simulink model "pod_elevation_model"  (R2021b)
settings: Solver=ode45  StartTime=0.0  StopTime=20  RelTol=1e-3
values from neighbouring files (symbols this model uses):
  fric_gear_motor_pod_elevation = 0.23125*0.42    (= 0.097125)    [loading_project.m]
  ts3 = 10^-3    (= 0.001)    [loading_project.m]
libraries: simulink x3, dspsrcs4 x1
settings Model: Creator=noait  LastModifiedBy=noait

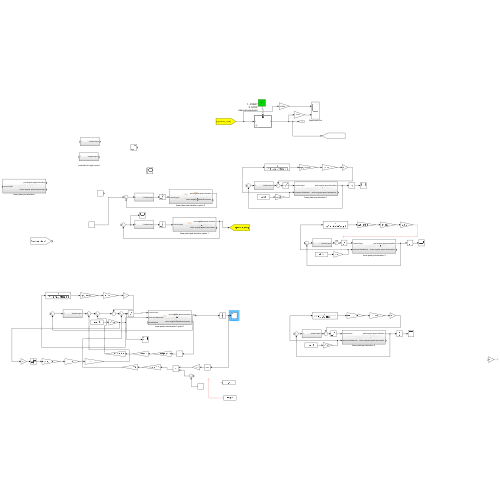
[thumbnail: Simulink's stored preview of the top-level diagram]
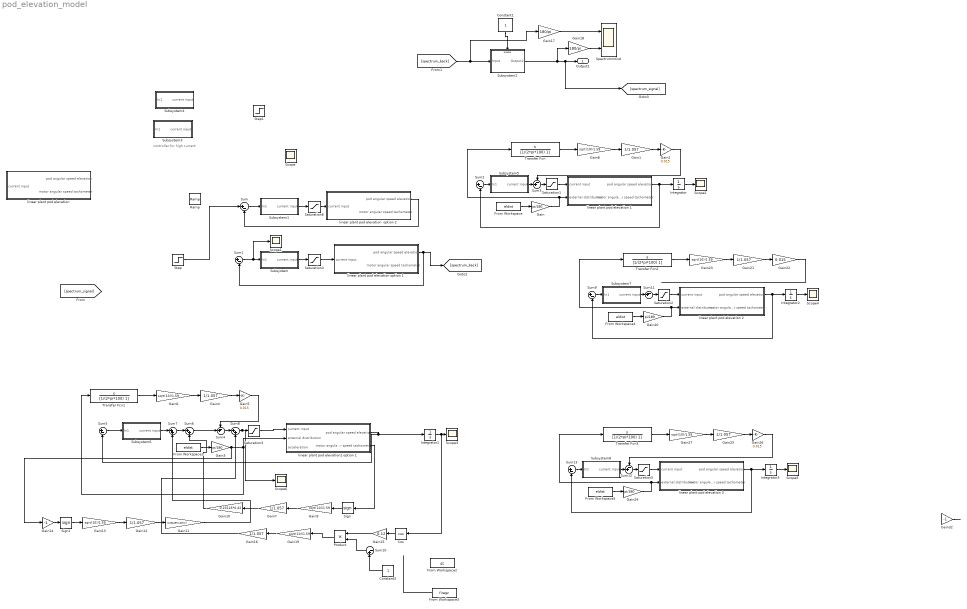
== system pod_elevation_model ==
  note: controller for high current
  Constant1 : Constant  OutDataTypeStr=boolean
      settings: AttributesFormatString=1 - START\n0 -STOP\ninternal spectrum
      settings: OpenFcn=|
      | if get_param(gcbh,'value')-48 set_param(gcbh,'value','0','backgroundcolor','red');
      | else set_param(gcbh,'value','1','backgroundcolor','green');
      | end
  Constant3 : Constant
  Cos : Trigonometry  Operator=cos
  From Workspace{,1,4..5} (4 alike) : FromWorkspace  VariableName=eldist  SampleTime=ts3/3  Interpolate=off  ZeroCross=off  OutputAfterFinalValue=Setting to zero
  From Workspace2 : FromWorkspace  VariableName=gz  SampleTime=ts3/3  Interpolate=off  ZeroCross=off  OutputAfterFinalValue=Setting to zero
  From Workspace3 : FromWorkspace  VariableName=firegz  SampleTime=ts3/9  Interpolate=off  ZeroCross=off  OutputAfterFinalValue=Setting to zero
  Gain{,3,20,24} (4 alike) : Gain  Gain=pi/180
  Gain{1,4,7,12,16,21,25} (7 alike) : Gain  Gain=1/1.057
  Gain10 : Gain  Gain=0.23125*0.42
  Gain11 : Gain  Gain=0.23125*0.42*0.7
  Gain{6,8..9,13,19,23,27} (7 alike) : Gain  Gain=sqrt(10)/1.59
  Gain14 : Gain  Gain=-1
  Gain15 : Gain  Gain=0.12
  Gain17 : Gain  Gain=180/pi
  Gain18 : Gain  Gain=180/pi
  Gain{2,5,22,26} (4 alike) : Gain  Gain=0.015
  Gain32 : Gain  Gain=-1
  Integrator{,1..3} (4 alike) : Integrator
  Product : Product
  Ramp : simulink/Sources/Ramp  slope=1  start=0  InitialOutput=0
  Saturation{1..2,4..5} (4 alike) : Saturate  UpperLimit=11.933*sqrt(10)/1.59  LowerLimit=-11.933*sqrt(10)/1.59  ZeroCross=off
  Saturation3 : Saturate  UpperLimit=11.933*sqrt(10)/1.59  LowerLimit=-11.933*sqrt(10)/1.59
  Saturation6 : Saturate  UpperLimit=11.933*sqrt(10)*0.5/(1.59*0.52)  LowerLimit=-11.933*sqrt(10)*0.5/(1.59*0.52)  ZeroCross=off
  Scope : Scope  NumInputPorts=2
  Scope{1..6} (6 alike) : Scope
  Sign : Signum
  Sign1 : Signum
  SpectrumInOut : Scope  NumInputPorts=2
  Step : Step  SampleTime=0  ZeroCross=off
  Step1 : Step  After=22  SampleTime=0
  Subsystem : Subsystem
  Subsystem1 : Subsystem
  Subsystem2 : Subsystem  mask{GAIN=0.1%2*pi/180%0.5*pi/180, InitFreq=1, TargetTime=500, FreqAtTime=500}
      mask prompts: InitFreq "INITIAL FREQUENCY"; TargetTime "Target Time"; FreqAtTime "Frequency at Time"
  Subsystem3 : Subsystem
  Subsystem4 : Subsystem
  Subsystem5 : Subsystem
  Subsystem6 : Subsystem
  Subsystem7 : Subsystem
  Subsystem8 : Subsystem
  Sum{,1..2,5,9,13} (6 alike) : Sum  Inputs=|+-
  Sum10 : Sum  Inputs=|-+
  Sum{3..4,11..12} (4 alike) : Sum  Inputs=-+|
  Sum6 : Sum  Inputs=|++
  Sum7 : Sum  Inputs=|++
  Sum8 : Sum  Inputs=|++
  Transfer Fcn{,1..3} (4 alike) : TransferFcn  Numerator=[1 0]  Denominator=[1/(2*pi*100) 1]
  "linear plant pod elevation " : Subsystem
  linear plant pod elevation  option 2 : Subsystem
  linear plant pod elevation 1 : Subsystem
  linear plant pod elevation 2 : Subsystem
  linear plant pod elevation 3 : Subsystem
  linear plant pod elevation option 1 : Subsystem
  linear plant pod elevation1 option 1 : Subsystem
  Output2 : Outport
  wires:
  Sum/1 -> Subsystem1/1(In1)
  Sum1/1 -> Scope1/1, Subsystem/1(In1)
  Saturation6/1 -> linear plant pod elevation  option 2/1(current input)
  Gain18/1 -> SpectrumInOut/2
  Gain17/1 -> SpectrumInOut/1
  [spectrum_back] -> Gain17/1, Subsystem2/1(Input)
  Subsystem2/1(Output2) -> [spectrum_signal], Output2/1, Gain18/1
  Constant1/1 -> Subsystem2/Enable
  Saturation4/1 -> linear plant pod elevation option 1/1(current input)
  linear plant pod elevation  option 2/1(pod angular speed elevation) -> Sum/2
  Subsystem1/1(current input) -> Saturation6/1
  linear plant pod elevation option 1/1(pod angular speed elevation) -> Sum1/2, [spectrum_back]
  Subsystem/1(current input) -> Saturation4/1
  Sum2/1 -> Subsystem5/1(In1)
  linear plant pod elevation 1/1(pod angular speed elevation) -> Integrator/1, Sum2/2
  Saturation1/1 -> linear plant pod elevation 1/1(current input)
  From Workspace/1 -> Gain/1
  Gain/1 -> Transfer Fcn/1, linear plant pod elevation 1/2(external distribution)
  Integrator/1 -> Scope2/1
  Gain8/1 -> Gain1/1
  Transfer Fcn/1 -> Gain8/1
  Gain1/1 -> Gain2/1
  Sum3/1 -> Saturation1/1
  Subsystem5/1(current input) -> Sum3/2
  Gain2/1 -> Sum3/1
  Saturation3/1 -> linear plant pod elevation1 option 1/1(current input)
  Sum5/1 -> Subsystem6/1(In1)
  linear plant pod elevation1 option 1/1(pod angular speed elevation) -> Integrator1/1, Sum5/2
  Integrator1/1 -> Cos/1, Scope3/1
  From Workspace1/1 -> Gain3/1
  Gain3/1 -> Gain14/1, linear plant pod elevation1 option 1/2(external distribution), Transfer Fcn1/1
  Gain4/1 -> Gain5/1
  Transfer Fcn1/1 -> Gain6/1
  Gain6/1 -> Gain4/1
  Gain5/1 -> Sum4/1
  linear plant pod elevation1 option 1/2("motor angular speed tachometer ") -> Sign/1
  Gain9/1 -> Gain7/1
  Sign/1 -> Gain9/1
  Gain7/1 -> Gain10/1
  Sum6/1 -> Sum4/2
  Gain10/1 -> Sum6/2
  Gain12/1 -> Gain11/1
  Sign1/1 -> Gain13/1
  Gain13/1 -> Gain12/1
  Subsystem6/1(current input) -> Sum7/1
  Sum7/1 -> Sum6/1
  Gain11/1 -> Sum7/2
  Cos/1 -> Gain15/1
  Sum4/1 -> Sum8/1
  Sum8/1 -> Scope6/1, Saturation3/1
  Gain19/1 -> Gain16/1
  Gain15/1 -> Product/1
  Product/1 -> Gain19/1
  Constant3/1 -> Sum10/2
  Sum10/1 -> Product/2
  From Workspace3/1 -> ?
  Gain21/1 -> Gain22/1
  Gain20/1 -> Transfer Fcn2/1, linear plant pod elevation 2/2(external distribution)
  From Workspace4/1 -> Gain20/1
  linear plant pod elevation 2/1(pod angular speed elevation) -> Integrator2/1, Sum9/2
  Integrator2/1 -> Scope4/1
  Transfer Fcn2/1 -> Gain23/1
  Sum11/1 -> Saturation2/1
  Gain23/1 -> Gain21/1
  Saturation2/1 -> linear plant pod elevation 2/1(current input)
  Sum9/1 -> Subsystem7/1(In1)
  Subsystem7/1(current input) -> Sum11/2
  Gain22/1 -> ?
  Gain14/1 -> Sign1/1
  Gain26/1 -> Sum12/1
  Sum12/1 -> Saturation5/1
  Gain27/1 -> Gain25/1
  From Workspace5/1 -> Gain24/1
  Integrator3/1 -> Scope5/1
  linear plant pod elevation 3/1(pod angular speed elevation) -> Integrator3/1, Sum13/2
  Gain25/1 -> Gain26/1
  Gain24/1 -> Transfer Fcn3/1, linear plant pod elevation 3/2(external distribution)
  Subsystem8/1(current input) -> Sum12/2
  Saturation5/1 -> linear plant pod elevation 3/1(current input)
  Sum13/1 -> Subsystem8/1(In1)
  Transfer Fcn3/1 -> Gain27/1
  Gain32/1 -> ?
  Step/1 -> Sum/1
  Gain16/1 -> Sum8/2

== system pod_elevation_model/Subsystem ==
  In1 : Inport
  Gain : Gain  Gain=85
  Gain4 : Gain  Gain=2*pi*3
  Gain5 : Gain
  Integrator1 : Integrator
  Sum2 : Sum  Inputs=|++
  current input : Outport
  wires:
  In1/1 -> Gain/1
  Integrator1/1 -> Sum2/1
  Gain4/1 -> Integrator1/1
  Gain/1 -> Gain4/1, Gain5/1
  Gain5/1 -> Sum2/2
  Sum2/1 -> current input/1

== system pod_elevation_model/Subsystem1 ==
  In1 : Inport
  Gain : Gain  Gain=150
  Gain4 : Gain  Gain=2*pi*1
  Gain5 : Gain
  Integrator1 : Integrator
  Sum2 : Sum  Inputs=|++
  current input : Outport
  wires:
  In1/1 -> Gain/1
  Integrator1/1 -> Sum2/1
  Gain4/1 -> Integrator1/1
  Gain/1 -> Gain4/1, Gain5/1
  Gain5/1 -> Sum2/2
  Sum2/1 -> current input/1

== system pod_elevation_model/Subsystem2 ==
  Input : Inport
  Enable : EnablePort  StatesWhenEnabling=reset
  Chirp : dspsrcs4/Chirp  sweep=Linear  mode=Unidirectional  f0=1  f1=160  t1=160  Tsweep=160  phase=0  Ts=1/1000  spf=1  datatype=Double  OutputFrames=off
  Chirp Signal : simulink/Sources/Chirp Signal  Commented=on  f1=InitFreq  T=TargetTime  f2=FreqAtTime
  Chirp Signal1 : simulink/Sources/Chirp Signal  f1=1  T=160  f2=160
  Mux2 : Mux  Inputs=2
  Scope2 : Scope
  TSABAD_out_log : Scope
  gain 3 : Gain  Gain=GAIN  SaturateOnIntegerOverflow=on  SampleTime=ts3/3  OutDataTypeStr=Inherit: Same as input  ParamDataTypeStr=Inherit: Same as input
  Output2 : Outport
  wires:
  gain 3/1 -> Output2/1, Mux2/1
  Chirp Signal/1 -> ?
  Input/1 -> Mux2/2
  Mux2/1 -> TSABAD_out_log/1
  Chirp Signal1/1 -> gain 3/1, Scope2/1

== system pod_elevation_model/Subsystem3 ==
  In1 : Inport
  Gain : Gain  Gain=85
  Gain4 : Gain  Gain=2*pi*0.5
  Gain5 : Gain
  Integrator1 : Integrator
  Sum2 : Sum  Inputs=|++
  current input : Outport
  wires:
  In1/1 -> Gain/1
  Integrator1/1 -> Sum2/1
  Gain4/1 -> Integrator1/1
  Gain/1 -> Gain4/1, Gain5/1
  Gain5/1 -> Sum2/2
  Sum2/1 -> current input/1

== system pod_elevation_model/Subsystem4 ==
  In1 : Inport
  Gain : Gain  Gain=85
  Gain4 : Gain  Gain=2*pi*0.5
  Gain5 : Gain
  Integrator1 : Integrator
  Sum2 : Sum  Inputs=|++
  current input : Outport
  wires:
  In1/1 -> Gain/1
  Integrator1/1 -> Sum2/1
  Gain4/1 -> Integrator1/1
  Gain/1 -> Gain4/1, Gain5/1
  Gain5/1 -> Sum2/2
  Sum2/1 -> current input/1

== system pod_elevation_model/Subsystem5 ==
  In1 : Inport
  Gain : Gain  Gain=85
  Gain4 : Gain  Gain=2*pi*3
  Gain5 : Gain
  Integrator1 : Integrator
  Sum2 : Sum  Inputs=|++
  current input : Outport
  wires:
  In1/1 -> Gain/1
  Integrator1/1 -> Sum2/1
  Gain4/1 -> Integrator1/1
  Gain/1 -> Gain4/1, Gain5/1
  Gain5/1 -> Sum2/2
  Sum2/1 -> current input/1

== system pod_elevation_model/Subsystem6 ==
  In1 : Inport
  Gain : Gain  Gain=150
  Gain4 : Gain  Gain=2*pi*1
  Gain5 : Gain
  Integrator1 : Integrator
  Sum2 : Sum  Inputs=|++
  current input : Outport
  wires:
  In1/1 -> Gain/1
  Integrator1/1 -> Sum2/1
  Gain4/1 -> Integrator1/1
  Gain/1 -> Gain4/1, Gain5/1
  Gain5/1 -> Sum2/2
  Sum2/1 -> current input/1

== system pod_elevation_model/Subsystem7 ==
  In1 : Inport
  Gain : Gain  Gain=85
  Gain4 : Gain  Gain=2*pi*3
  Gain5 : Gain
  Integrator1 : Integrator
  Sum2 : Sum  Inputs=|++
  current input : Outport
  wires:
  In1/1 -> Gain/1
  Integrator1/1 -> Sum2/1
  Gain4/1 -> Integrator1/1
  Gain/1 -> Gain4/1, Gain5/1
  Gain5/1 -> Sum2/2
  Sum2/1 -> current input/1

== system pod_elevation_model/Subsystem8 ==
  In1 : Inport
  Gain : Gain  Gain=85
  Gain4 : Gain  Gain=2*pi*3
  Gain5 : Gain
  Integrator1 : Integrator
  Sum2 : Sum  Inputs=|++
  current input : Outport
  wires:
  In1/1 -> Gain/1
  Integrator1/1 -> Sum2/1
  Gain4/1 -> Integrator1/1
  Gain/1 -> Gain4/1, Gain5/1
  Gain5/1 -> Sum2/2
  Sum2/1 -> current input/1

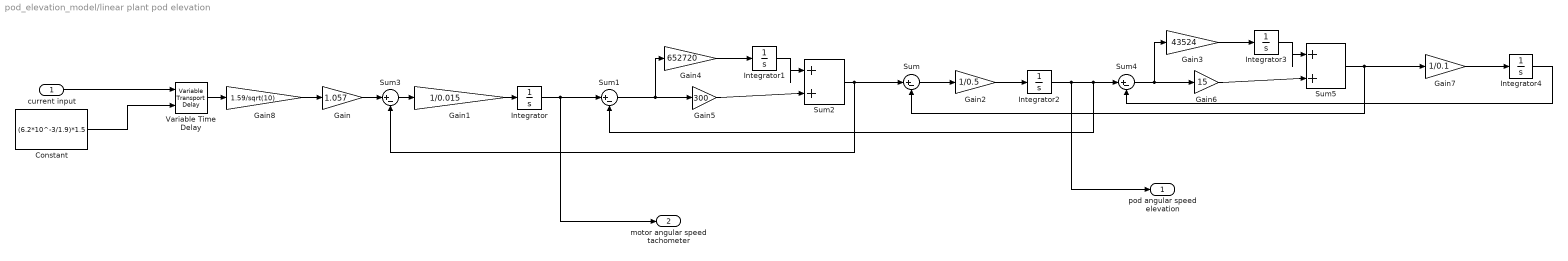
== system pod_elevation_model/linear plant pod elevation  ==
  current input : Inport
  Constant : Constant  Value=(6.2*10^-3/1.9)*1.5  SampleTime=-1
  Gain : Gain  Gain=1.057
  Gain1 : Gain  Gain=1/0.015
  Gain2 : Gain  Gain=1/0.5
  Gain3 : Gain  Gain=43524
  Gain4 : Gain  Gain=652720
  Gain5 : Gain  Gain=300
  Gain6 : Gain  Gain=15
  Gain7 : Gain  Gain=1/0.1
  Gain8 : Gain  Gain=1.59/sqrt(10)
  Integrator{,1..4} (5 alike) : Integrator
  Sum{,1,3..4} (4 alike) : Sum  Inputs=|+-
  Sum2 : Sum  Inputs=|++
  Sum5 : Sum  Inputs=|++
  Variable Time Delay : VariableTransportDelay  MaximumDelay=10  TransDelayFeedthrough=on
  pod angular speed elevation : Outport
  "motor angular speed tachometer " : Outport  Port=2
  wires:
  Integrator3/1 -> Sum5/1
  Gain7/1 -> Integrator4/1
  Gain8/1 -> Gain/1
  Sum5/1 -> Gain7/1, Sum/2
  Gain6/1 -> Sum5/2
  Sum/1 -> Gain2/1
  Gain5/1 -> Sum2/2
  Integrator4/1 -> Sum4/2
  Gain/1 -> Sum3/1
  Sum1/1 -> Gain5/1, Gain4/1
  Sum4/1 -> Gain6/1, Gain3/1
  Integrator1/1 -> Sum2/1
  Variable Time Delay/1 -> Gain8/1
  Constant/1 -> Variable Time Delay/2
  Sum3/1 -> Gain1/1
  Integrator2/1 -> pod angular speed elevation/1, Sum1/2, Sum4/1
  Sum2/1 -> Sum/1, Sum3/2
  Gain2/1 -> Integrator2/1
  Gain4/1 -> Integrator1/1
  Gain3/1 -> Integrator3/1
  Integrator/1 -> "motor angular speed tachometer "/1, Sum1/1
  Gain1/1 -> Integrator/1
  current input/1 -> Variable Time Delay/1

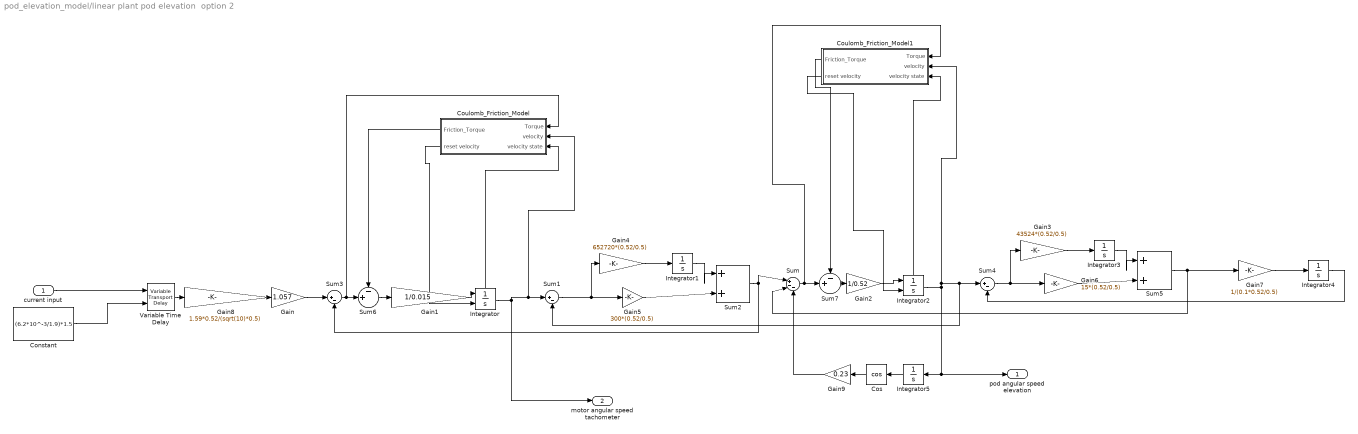
== system pod_elevation_model/linear plant pod elevation  option 2 ==
  current input : Inport
  Constant : Constant  Value=(6.2*10^-3/1.9)*1.5  SampleTime=-1
  Cos : Trigonometry  Operator=cos
  Coulomb_Friction_Model : Subsystem
  Coulomb_Friction_Model1 : Subsystem
  Gain : Gain  Gain=1.057
  Gain1 : Gain  Gain=1/0.015
  Gain2 : Gain  Gain=1/0.52
  Gain3 : Gain  Gain=43524*(0.52/0.5)
  Gain4 : Gain  Gain=652720*(0.52/0.5)
  Gain5 : Gain  Gain=300*(0.52/0.5)
  Gain6 : Gain  Gain=15*(0.52/0.5)
  Gain7 : Gain  Gain=1/(0.1*0.52/0.5)
  Gain8 : Gain  Gain=1.59*0.52/(sqrt(10)*0.5)
  Gain9 : Gain  Gain=0.23
  Integrator : Integrator  ExternalReset=rising  ShowStatePort=on  ZeroCross=off
  Integrator{1,3..5} (4 alike) : Integrator
  Integrator2 : Integrator  ExternalReset=rising  ShowStatePort=on  ZeroCross=off
  Sum : Sum  Inputs=|+--
  Sum1 : Sum  Inputs=|+-
  Sum2 : Sum  Inputs=|++
  Sum3 : Sum  Inputs=|+-
  Sum4 : Sum  Inputs=|+-
  Sum5 : Sum  Inputs=|++
  Sum6 : Sum  Inputs=-+|
  Sum7 : Sum  Inputs=-+|
  Variable Time Delay : VariableTransportDelay  MaximumDelay=10  TransDelayFeedthrough=on
  pod angular speed elevation : Outport
  "motor angular speed tachometer " : Outport  Port=2
  wires:
  Integrator3/1 -> Sum5/1
  Gain7/1 -> Integrator4/1
  Gain8/1 -> Gain/1
  Sum5/1 -> Gain7/1, Sum/2
  Gain6/1 -> Sum5/2
  Gain5/1 -> Sum2/2
  Integrator4/1 -> Sum4/2
  Gain/1 -> Sum3/1
  Sum1/1 -> Gain5/1, Gain4/1
  Sum4/1 -> Gain6/1, Gain3/1
  Integrator1/1 -> Sum2/1
  current input/1 -> Variable Time Delay/1
  Variable Time Delay/1 -> Gain8/1
  Constant/1 -> Variable Time Delay/2
  Sum2/1 -> Sum/1, Sum3/2
  Gain2/1 -> Integrator2/1
  Gain4/1 -> Integrator1/1
  Gain3/1 -> Integrator3/1
  Gain1/1 -> Integrator/1
  Integrator/1 -> Coulomb_Friction_Model/2(velocity), Sum1/1, "motor angular speed tachometer "/1
  Coulomb_Friction_Model/2(reset velocity) -> Integrator/2
  Sum3/1 -> Coulomb_Friction_Model/1(Torque), Sum6/2
  Integrator/State -> Coulomb_Friction_Model/3(velocity state)
  Coulomb_Friction_Model/1(Friction_Torque) -> Sum6/1
  Sum6/1 -> Gain1/1
  Integrator5/1 -> Cos/1
  Cos/1 -> Gain9/1
  Gain9/1 -> Sum/3
  Sum/1 -> Coulomb_Friction_Model1/1(Torque), Sum7/2
  Integrator2/State -> Coulomb_Friction_Model1/3(velocity state)
  Coulomb_Friction_Model1/1(Friction_Torque) -> Sum7/1
  Coulomb_Friction_Model1/2(reset velocity) -> Integrator2/2
  Integrator2/1 -> Coulomb_Friction_Model1/2(velocity), Sum1/2, Sum4/1, Integrator5/1, pod angular speed elevation/1
  Sum7/1 -> Gain2/1

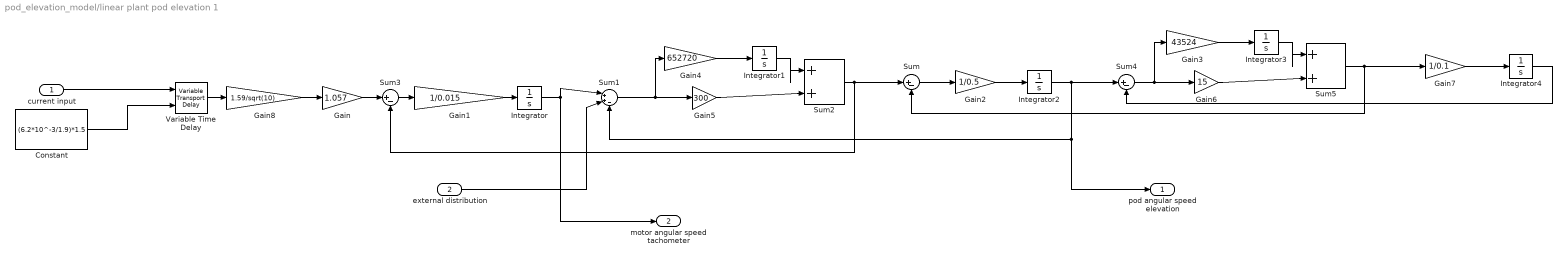
== system pod_elevation_model/linear plant pod elevation 1 ==
  current input : Inport
  external distribution : Inport  Port=2
  Constant : Constant  Value=(6.2*10^-3/1.9)*1.5  SampleTime=-1
  Gain : Gain  Gain=1.057
  Gain1 : Gain  Gain=1/0.015
  Gain2 : Gain  Gain=1/0.5
  Gain3 : Gain  Gain=43524
  Gain4 : Gain  Gain=652720
  Gain5 : Gain  Gain=300
  Gain6 : Gain  Gain=15
  Gain7 : Gain  Gain=1/0.1
  Gain8 : Gain  Gain=1.59/sqrt(10)
  Integrator{,1..4} (5 alike) : Integrator
  Sum : Sum  Inputs=|+-
  Sum1 : Sum  Inputs=|++-
  Sum2 : Sum  Inputs=|++
  Sum3 : Sum  Inputs=|+-
  Sum4 : Sum  Inputs=|+-
  Sum5 : Sum  Inputs=|++
  Variable Time Delay : VariableTransportDelay  MaximumDelay=10  TransDelayFeedthrough=on
  pod angular speed elevation : Outport
  "motor angular speed tachometer " : Outport  Port=2
  wires:
  Integrator3/1 -> Sum5/1
  Gain7/1 -> Integrator4/1
  Gain8/1 -> Gain/1
  Sum5/1 -> Gain7/1, Sum/2
  Gain6/1 -> Sum5/2
  Sum/1 -> Gain2/1
  Gain5/1 -> Sum2/2
  Integrator4/1 -> Sum4/2
  Gain/1 -> Sum3/1
  Sum1/1 -> Gain5/1, Gain4/1
  Sum4/1 -> Gain6/1, Gain3/1
  Integrator1/1 -> Sum2/1
  Variable Time Delay/1 -> Gain8/1
  Constant/1 -> Variable Time Delay/2
  Sum3/1 -> Gain1/1
  Integrator2/1 -> Sum1/3, pod angular speed elevation/1, Sum4/1
  Sum2/1 -> Sum/1, Sum3/2
  Gain2/1 -> Integrator2/1
  Gain4/1 -> Integrator1/1
  Gain3/1 -> Integrator3/1
  Integrator/1 -> "motor angular speed tachometer "/1, Sum1/1
  Gain1/1 -> Integrator/1
  current input/1 -> Variable Time Delay/1
  external distribution/1 -> Sum1/2

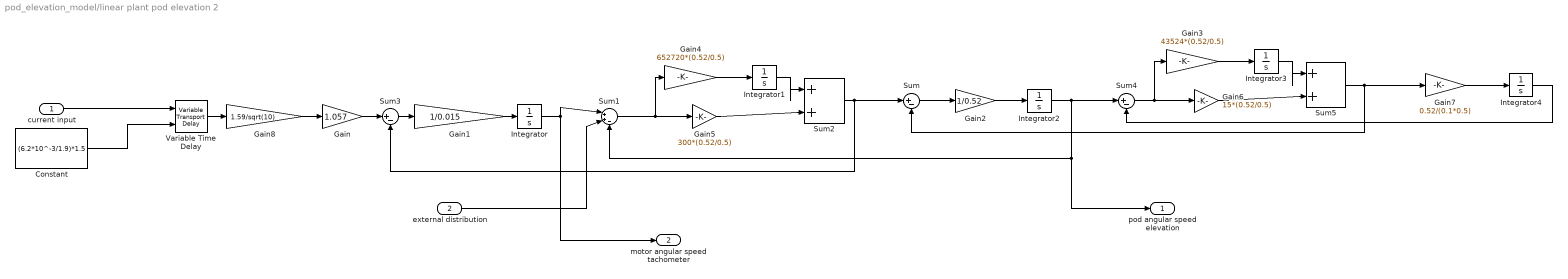
== system pod_elevation_model/linear plant pod elevation 2 ==
  current input : Inport
  external distribution : Inport  Port=2
  Constant : Constant  Value=(6.2*10^-3/1.9)*1.5  SampleTime=-1
  Gain : Gain  Gain=1.057
  Gain1 : Gain  Gain=1/0.015
  Gain2 : Gain  Gain=1/0.52
  Gain3 : Gain  Gain=43524*(0.52/0.5)
  Gain4 : Gain  Gain=652720*(0.52/0.5)
  Gain5 : Gain  Gain=300*(0.52/0.5)
  Gain6 : Gain  Gain=15*(0.52/0.5)
  Gain7 : Gain  Gain=0.52/(0.1*0.5)
  Gain8 : Gain  Gain=1.59/sqrt(10)
  Integrator{,1..4} (5 alike) : Integrator
  Sum : Sum  Inputs=|+-
  Sum1 : Sum  Inputs=|++-
  Sum2 : Sum  Inputs=|++
  Sum3 : Sum  Inputs=|+-
  Sum4 : Sum  Inputs=|+-
  Sum5 : Sum  Inputs=|++
  Variable Time Delay : VariableTransportDelay  MaximumDelay=10  TransDelayFeedthrough=on
  pod angular speed elevation : Outport
  "motor angular speed tachometer " : Outport  Port=2
  wires:
  Integrator3/1 -> Sum5/1
  Gain7/1 -> Integrator4/1
  Gain8/1 -> Gain/1
  Sum5/1 -> Gain7/1, Sum/2
  Gain6/1 -> Sum5/2
  Sum/1 -> Gain2/1
  Gain5/1 -> Sum2/2
  Integrator4/1 -> Sum4/2
  Gain/1 -> Sum3/1
  Sum1/1 -> Gain5/1, Gain4/1
  Sum4/1 -> Gain6/1, Gain3/1
  Integrator1/1 -> Sum2/1
  Variable Time Delay/1 -> Gain8/1
  Constant/1 -> Variable Time Delay/2
  Sum3/1 -> Gain1/1
  Integrator2/1 -> Sum1/3, pod angular speed elevation/1, Sum4/1
  Sum2/1 -> Sum/1, Sum3/2
  Gain2/1 -> Integrator2/1
  Gain4/1 -> Integrator1/1
  Gain3/1 -> Integrator3/1
  Integrator/1 -> "motor angular speed tachometer "/1, Sum1/1
  Gain1/1 -> Integrator/1
  current input/1 -> Variable Time Delay/1
  external distribution/1 -> Sum1/2

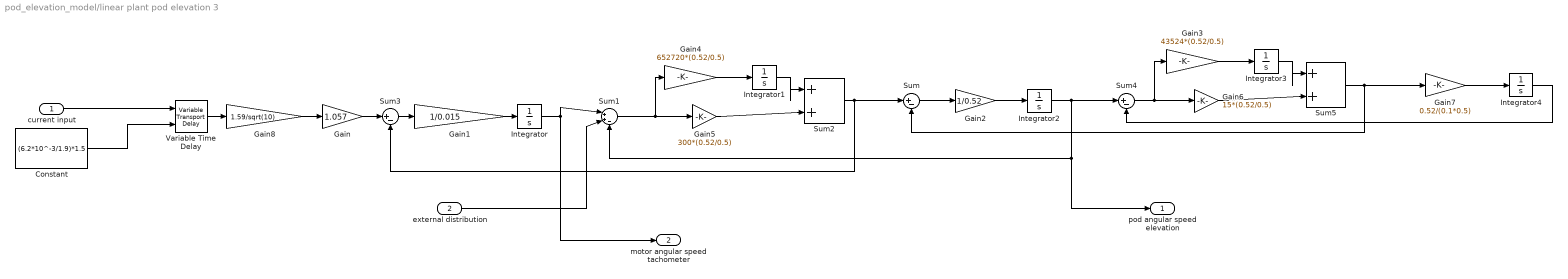
== system pod_elevation_model/linear plant pod elevation 3 ==
  current input : Inport
  external distribution : Inport  Port=2
  Constant : Constant  Value=(6.2*10^-3/1.9)*1.5  SampleTime=-1
  Gain : Gain  Gain=1.057
  Gain1 : Gain  Gain=1/0.015
  Gain2 : Gain  Gain=1/0.52
  Gain3 : Gain  Gain=43524*(0.52/0.5)
  Gain4 : Gain  Gain=652720*(0.52/0.5)
  Gain5 : Gain  Gain=300*(0.52/0.5)
  Gain6 : Gain  Gain=15*(0.52/0.5)
  Gain7 : Gain  Gain=0.52/(0.1*0.5)
  Gain8 : Gain  Gain=1.59/sqrt(10)
  Integrator{,1..4} (5 alike) : Integrator
  Sum : Sum  Inputs=|+-
  Sum1 : Sum  Inputs=|++-
  Sum2 : Sum  Inputs=|++
  Sum3 : Sum  Inputs=|+-
  Sum4 : Sum  Inputs=|+-
  Sum5 : Sum  Inputs=|++
  Variable Time Delay : VariableTransportDelay  MaximumDelay=10  TransDelayFeedthrough=on
  pod angular speed elevation : Outport
  "motor angular speed tachometer " : Outport  Port=2
  wires:
  Integrator3/1 -> Sum5/1
  Gain7/1 -> Integrator4/1
  Gain8/1 -> Gain/1
  Sum5/1 -> Gain7/1, Sum/2
  Gain6/1 -> Sum5/2
  Sum/1 -> Gain2/1
  Gain5/1 -> Sum2/2
  Integrator4/1 -> Sum4/2
  Gain/1 -> Sum3/1
  Sum1/1 -> Gain5/1, Gain4/1
  Sum4/1 -> Gain6/1, Gain3/1
  Integrator1/1 -> Sum2/1
  Variable Time Delay/1 -> Gain8/1
  Constant/1 -> Variable Time Delay/2
  Sum3/1 -> Gain1/1
  Integrator2/1 -> Sum1/3, pod angular speed elevation/1, Sum4/1
  Sum2/1 -> Sum/1, Sum3/2
  Gain2/1 -> Integrator2/1
  Gain4/1 -> Integrator1/1
  Gain3/1 -> Integrator3/1
  Integrator/1 -> "motor angular speed tachometer "/1, Sum1/1
  Gain1/1 -> Integrator/1
  current input/1 -> Variable Time Delay/1
  external distribution/1 -> Sum1/2

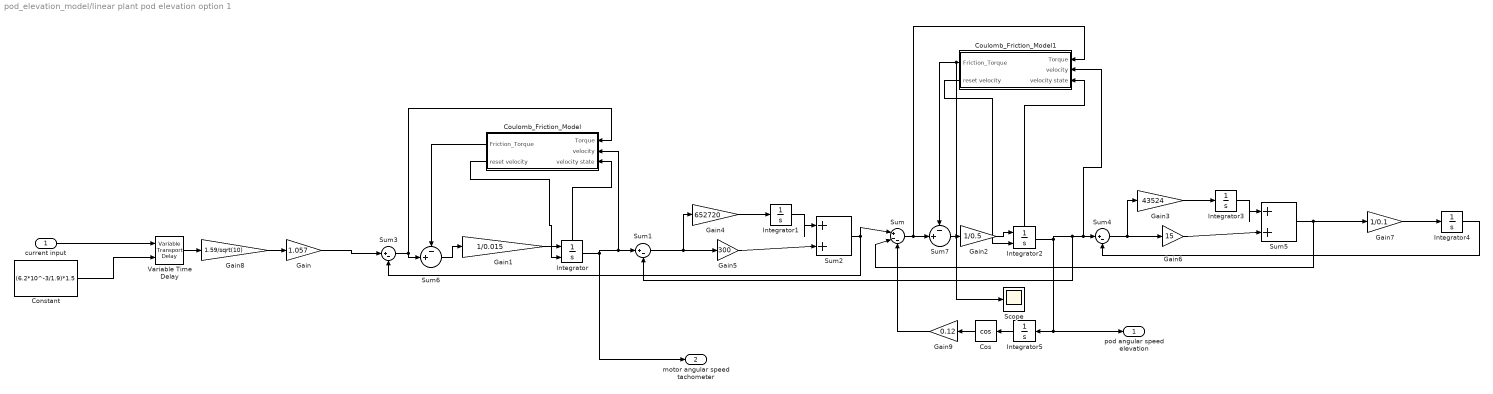
== system pod_elevation_model/linear plant pod elevation option 1 ==
  current input : Inport
  Constant : Constant  Value=(6.2*10^-3/1.9)*1.5  SampleTime=-1
  Cos : Trigonometry  Operator=cos
  Coulomb_Friction_Model : Subsystem
  Coulomb_Friction_Model1 : Subsystem
  Gain : Gain  Gain=1.057
  Gain1 : Gain  Gain=1/0.015
  Gain2 : Gain  Gain=1/0.5
  Gain3 : Gain  Gain=43524
  Gain4 : Gain  Gain=652720
  Gain5 : Gain  Gain=300
  Gain6 : Gain  Gain=15
  Gain7 : Gain  Gain=1/0.1
  Gain8 : Gain  Gain=1.59/sqrt(10)
  Gain9 : Gain  Gain=0.12
  Integrator : Integrator  ExternalReset=rising  ShowStatePort=on  ZeroCross=off
  Integrator{1,3..5} (4 alike) : Integrator
  Integrator2 : Integrator  ExternalReset=rising  ShowStatePort=on  ZeroCross=off
  Scope : Scope
  Sum : Sum  Inputs=|+--
  Sum1 : Sum  Inputs=|+-
  Sum2 : Sum  Inputs=|++
  Sum3 : Sum  Inputs=|+-
  Sum4 : Sum  Inputs=|+-
  Sum5 : Sum  Inputs=|++
  Sum6 : Sum  Inputs=-+|
  Sum7 : Sum  Inputs=-+|
  Variable Time Delay : VariableTransportDelay  MaximumDelay=10  TransDelayFeedthrough=on
  pod angular speed elevation : Outport
  "motor angular speed tachometer " : Outport  Port=2
  wires:
  Integrator3/1 -> Sum5/1
  Gain7/1 -> Integrator4/1
  Gain8/1 -> Gain/1
  Sum5/1 -> Gain7/1, Sum/2
  Gain6/1 -> Sum5/2
  Gain5/1 -> Sum2/2
  Integrator4/1 -> Sum4/2
  Gain/1 -> Sum3/1
  Sum1/1 -> Gain5/1, Gain4/1
  Sum4/1 -> Gain6/1, Gain3/1
  Integrator1/1 -> Sum2/1
  current input/1 -> Variable Time Delay/1
  Variable Time Delay/1 -> Gain8/1
  Constant/1 -> Variable Time Delay/2
  Sum2/1 -> Sum3/2, Sum/1
  Gain2/1 -> Integrator2/1
  Gain4/1 -> Integrator1/1
  Gain3/1 -> Integrator3/1
  Gain1/1 -> Integrator/1
  Integrator/1 -> Coulomb_Friction_Model/2(velocity), Sum1/1, "motor angular speed tachometer "/1
  Integrator/State -> Coulomb_Friction_Model/3(velocity state)
  Coulomb_Friction_Model/1(Friction_Torque) -> Sum6/1
  Sum3/1 -> Coulomb_Friction_Model/1(Torque), Sum6/2
  Coulomb_Friction_Model/2(reset velocity) -> Integrator/2
  Sum6/1 -> Gain1/1
  Gain9/1 -> Sum/3
  Integrator5/1 -> Cos/1
  Cos/1 -> Gain9/1
  Coulomb_Friction_Model1/1(Friction_Torque) -> Sum7/1, Scope/1
  Sum/1 -> Sum7/2, Coulomb_Friction_Model1/1(Torque)
  Integrator2/1 -> Sum1/2, Coulomb_Friction_Model1/2(velocity), Sum4/1, Integrator5/1, pod angular speed elevation/1
  Integrator2/State -> Coulomb_Friction_Model1/3(velocity state)
  Coulomb_Friction_Model1/2(reset velocity) -> Integrator2/2
  Sum7/1 -> Gain2/1

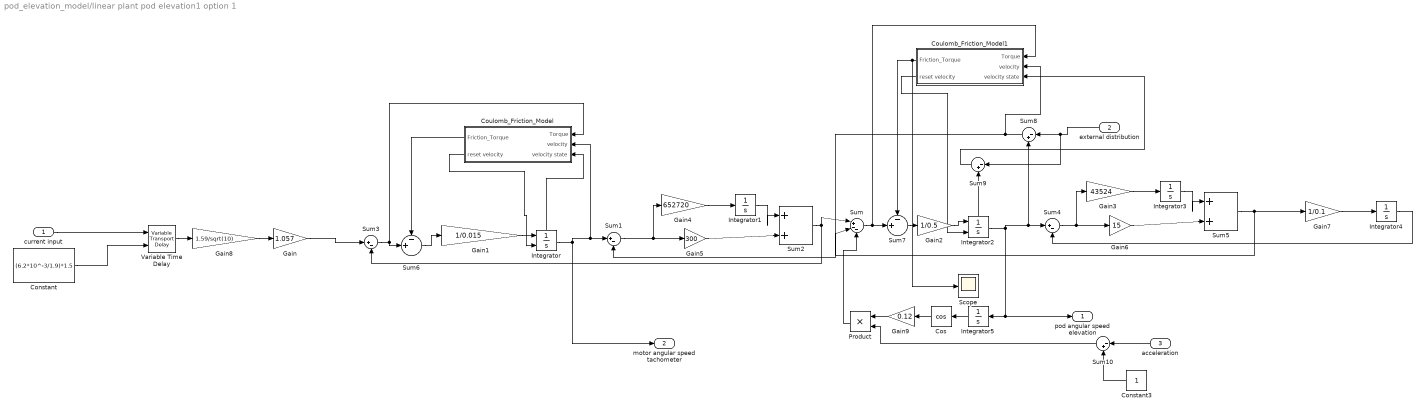
== system pod_elevation_model/linear plant pod elevation1 option 1 ==
  current input : Inport
  external distribution : Inport  Port=2
  acceleration : Inport  Port=3
  Constant : Constant  Value=(6.2*10^-3/1.9)*1.5  SampleTime=-1
  Constant3 : Constant
  Cos : Trigonometry  Operator=cos
  Coulomb_Friction_Model : Subsystem
  Coulomb_Friction_Model1 : Subsystem
  Gain : Gain  Gain=1.057
  Gain1 : Gain  Gain=1/0.015
  Gain2 : Gain  Gain=1/0.5
  Gain3 : Gain  Gain=43524
  Gain4 : Gain  Gain=652720
  Gain5 : Gain  Gain=300
  Gain6 : Gain  Gain=15
  Gain7 : Gain  Gain=1/0.1
  Gain8 : Gain  Gain=1.59/sqrt(10)
  Gain9 : Gain  Gain=0.12
  Integrator : Integrator  ExternalReset=rising  ShowStatePort=on  ZeroCross=off
  Integrator{1,3..5} (4 alike) : Integrator
  Integrator2 : Integrator  ExternalReset=rising  ShowStatePort=on  ZeroCross=off
  Product : Product
  Scope : Scope
  Sum : Sum  Inputs=|+--
  Sum1 : Sum  Inputs=|+-
  Sum10 : Sum  Inputs=|-+
  Sum2 : Sum  Inputs=|++
  Sum3 : Sum  Inputs=|+-
  Sum4 : Sum  Inputs=|+-
  Sum5 : Sum  Inputs=|++
  Sum6 : Sum  Inputs=-+|
  Sum7 : Sum  Inputs=-+|
  Sum8 : Sum  Inputs=|-+
  Sum9 : Sum  Inputs=|-+
  Variable Time Delay : VariableTransportDelay  MaximumDelay=10  TransDelayFeedthrough=on
  pod angular speed elevation : Outport
  "motor angular speed tachometer " : Outport  Port=2
  wires:
  Integrator3/1 -> Sum5/1
  Gain7/1 -> Integrator4/1
  Gain8/1 -> Gain/1
  Sum5/1 -> Gain7/1, Sum/2
  Gain6/1 -> Sum5/2
  Gain5/1 -> Sum2/2
  Integrator4/1 -> Sum4/2
  Gain/1 -> Sum3/1
  Sum1/1 -> Gain5/1, Gain4/1
  Sum4/1 -> Gain6/1, Gain3/1
  Integrator1/1 -> Sum2/1
  current input/1 -> Variable Time Delay/1
  Variable Time Delay/1 -> Gain8/1
  Constant/1 -> Variable Time Delay/2
  Sum2/1 -> Sum3/2, Sum/1
  Gain2/1 -> Integrator2/1
  Gain4/1 -> Integrator1/1
  Gain3/1 -> Integrator3/1
  Gain1/1 -> Integrator/1
  Integrator/1 -> Coulomb_Friction_Model/2(velocity), Sum1/1, "motor angular speed tachometer "/1
  Integrator/State -> Coulomb_Friction_Model/3(velocity state)
  Coulomb_Friction_Model/1(Friction_Torque) -> Sum6/1
  Sum3/1 -> Coulomb_Friction_Model/1(Torque), Sum6/2
  Coulomb_Friction_Model/2(reset velocity) -> Integrator/2
  Sum6/1 -> Gain1/1
  Integrator5/1 -> Cos/1
  Cos/1 -> Gain9/1
  Coulomb_Friction_Model1/1(Friction_Torque) -> Sum7/1, Scope/1
  Sum/1 -> Sum7/2, Coulomb_Friction_Model1/1(Torque)
  Integrator2/1 -> Sum8/2, Sum4/1, Integrator5/1, pod angular speed elevation/1
  Coulomb_Friction_Model1/2(reset velocity) -> Integrator2/2
  Sum7/1 -> Gain2/1
  external distribution/1 -> Sum9/1, Sum8/1
  Sum8/1 -> Sum1/2, Coulomb_Friction_Model1/2(velocity)
  Integrator2/State -> Sum9/2
  Sum9/1 -> Coulomb_Friction_Model1/3(velocity state)
  acceleration/1 -> Sum10/1
  Constant3/1 -> Sum10/2
  Sum10/1 -> Product/2
  Gain9/1 -> Product/1
  Product/1 -> Sum/3

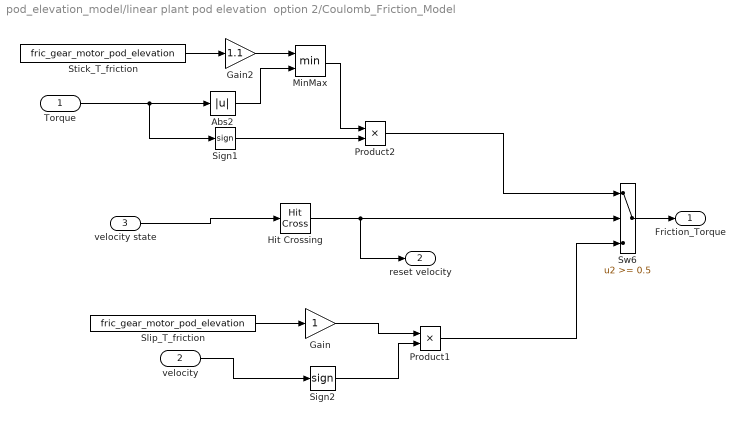
== system pod_elevation_model/linear plant pod elevation  option 2/Coulomb_Friction_Model ==
  Torque : Inport
  velocity : Inport  Port=2
  velocity state : Inport  Port=3
  Abs2 : Abs  ZeroCross=off
  Gain : Gain
  Gain2 : Gain  Gain=1.1
  Hit Crossing : HitCross  ZeroCross=off
  MinMax : MinMax  Inputs=2
  Product1 : Product  RndMeth=Zero
  Product2 : Product  RndMeth=Zero
  Sign1 : Signum  ZeroCross=off
  Sign2 : Signum  ZeroCross=off
  Slip_T_friction : Constant  Value=fric_gear_motor_pod_elevation
  Stick_T_friction : Constant  Value=fric_gear_motor_pod_elevation
  Sw6 : Switch  Threshold=0.5  ZeroCross=off  SaturateOnIntegerOverflow=on  InputSameDT=on
  Friction_Torque : Outport
  reset velocity : Outport  Port=2
  wires:
  Torque/1 -> Sign1/1, Abs2/1
  Sw6/1 -> Friction_Torque/1
  Hit Crossing/1 -> reset velocity/1, Sw6/2
  Abs2/1 -> MinMax/2
  MinMax/1 -> Product2/1
  Product2/1 -> Sw6/1
  Product1/1 -> Sw6/3
  Stick_T_friction/1 -> Gain2/1
  Gain2/1 -> MinMax/1
  Sign2/1 -> Product1/2
  velocity/1 -> Sign2/1
  Sign1/1 -> Product2/2
  velocity state/1 -> Hit Crossing/1
  Slip_T_friction/1 -> Gain/1
  Gain/1 -> Product1/1

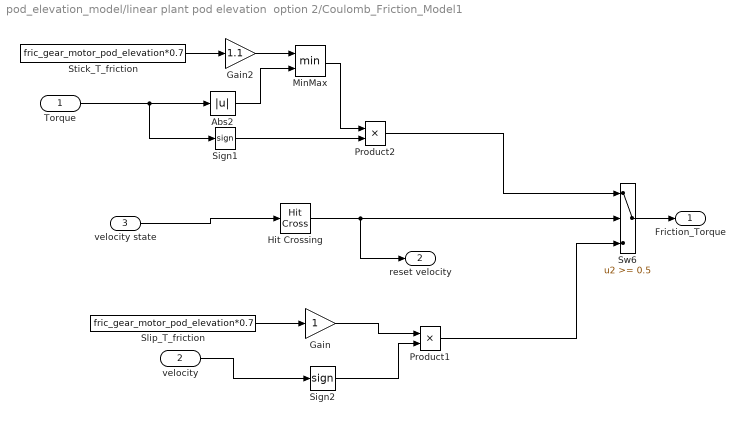
== system pod_elevation_model/linear plant pod elevation  option 2/Coulomb_Friction_Model1 ==
  Torque : Inport
  velocity : Inport  Port=2
  velocity state : Inport  Port=3
  Abs2 : Abs  ZeroCross=off
  Gain : Gain
  Gain2 : Gain  Gain=1.1
  Hit Crossing : HitCross  ZeroCross=off
  MinMax : MinMax  Inputs=2
  Product1 : Product  RndMeth=Zero
  Product2 : Product  RndMeth=Zero
  Sign1 : Signum  ZeroCross=off
  Sign2 : Signum  ZeroCross=off
  Slip_T_friction : Constant  Value=fric_gear_motor_pod_elevation*0.7
  Stick_T_friction : Constant  Value=fric_gear_motor_pod_elevation*0.7
  Sw6 : Switch  Threshold=0.5  ZeroCross=off  SaturateOnIntegerOverflow=on  InputSameDT=on
  Friction_Torque : Outport
  reset velocity : Outport  Port=2
  wires:
  Torque/1 -> Sign1/1, Abs2/1
  Sw6/1 -> Friction_Torque/1
  Hit Crossing/1 -> reset velocity/1, Sw6/2
  Abs2/1 -> MinMax/2
  MinMax/1 -> Product2/1
  Product2/1 -> Sw6/1
  Product1/1 -> Sw6/3
  Stick_T_friction/1 -> Gain2/1
  Gain2/1 -> MinMax/1
  Sign2/1 -> Product1/2
  velocity/1 -> Sign2/1
  Sign1/1 -> Product2/2
  velocity state/1 -> Hit Crossing/1
  Slip_T_friction/1 -> Gain/1
  Gain/1 -> Product1/1

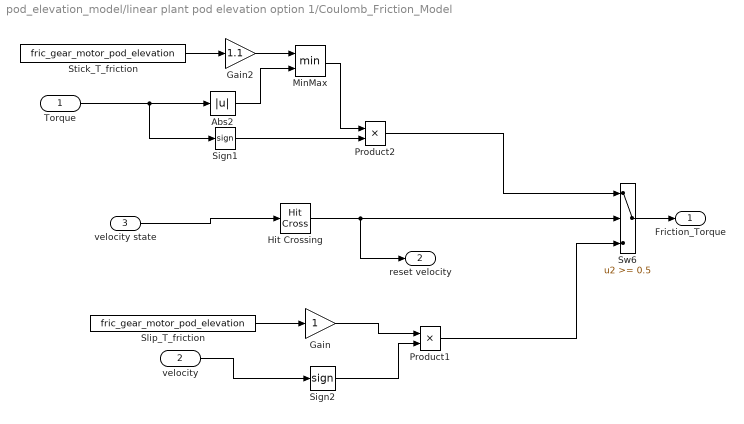
== system pod_elevation_model/linear plant pod elevation option 1/Coulomb_Friction_Model ==
  Torque : Inport
  velocity : Inport  Port=2
  velocity state : Inport  Port=3
  Abs2 : Abs  ZeroCross=off
  Gain : Gain
  Gain2 : Gain  Gain=1.1
  Hit Crossing : HitCross  ZeroCross=off
  MinMax : MinMax  Inputs=2
  Product1 : Product  RndMeth=Zero
  Product2 : Product  RndMeth=Zero
  Sign1 : Signum  ZeroCross=off
  Sign2 : Signum  ZeroCross=off
  Slip_T_friction : Constant  Value=fric_gear_motor_pod_elevation
  Stick_T_friction : Constant  Value=fric_gear_motor_pod_elevation
  Sw6 : Switch  Threshold=0.5  ZeroCross=off  SaturateOnIntegerOverflow=on  InputSameDT=on
  Friction_Torque : Outport
  reset velocity : Outport  Port=2
  wires:
  Torque/1 -> Sign1/1, Abs2/1
  Sw6/1 -> Friction_Torque/1
  Hit Crossing/1 -> reset velocity/1, Sw6/2
  Abs2/1 -> MinMax/2
  MinMax/1 -> Product2/1
  Product2/1 -> Sw6/1
  Product1/1 -> Sw6/3
  Stick_T_friction/1 -> Gain2/1
  Gain2/1 -> MinMax/1
  Sign2/1 -> Product1/2
  velocity/1 -> Sign2/1
  Sign1/1 -> Product2/2
  velocity state/1 -> Hit Crossing/1
  Slip_T_friction/1 -> Gain/1
  Gain/1 -> Product1/1

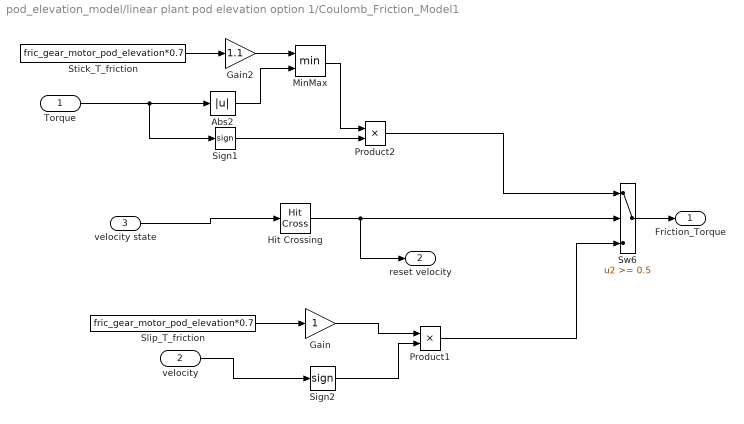
== system pod_elevation_model/linear plant pod elevation option 1/Coulomb_Friction_Model1 ==
  Torque : Inport
  velocity : Inport  Port=2
  velocity state : Inport  Port=3
  Abs2 : Abs  ZeroCross=off
  Gain : Gain
  Gain2 : Gain  Gain=1.1
  Hit Crossing : HitCross  ZeroCross=off
  MinMax : MinMax  Inputs=2
  Product1 : Product  RndMeth=Zero
  Product2 : Product  RndMeth=Zero
  Sign1 : Signum  ZeroCross=off
  Sign2 : Signum  ZeroCross=off
  Slip_T_friction : Constant  Value=fric_gear_motor_pod_elevation*0.7
  Stick_T_friction : Constant  Value=fric_gear_motor_pod_elevation*0.7
  Sw6 : Switch  Threshold=0.5  ZeroCross=off  SaturateOnIntegerOverflow=on  InputSameDT=on
  Friction_Torque : Outport
  reset velocity : Outport  Port=2
  wires:
  Torque/1 -> Sign1/1, Abs2/1
  Sw6/1 -> Friction_Torque/1
  Hit Crossing/1 -> reset velocity/1, Sw6/2
  Abs2/1 -> MinMax/2
  MinMax/1 -> Product2/1
  Product2/1 -> Sw6/1
  Product1/1 -> Sw6/3
  Stick_T_friction/1 -> Gain2/1
  Gain2/1 -> MinMax/1
  Sign2/1 -> Product1/2
  velocity/1 -> Sign2/1
  Sign1/1 -> Product2/2
  velocity state/1 -> Hit Crossing/1
  Slip_T_friction/1 -> Gain/1
  Gain/1 -> Product1/1

== system pod_elevation_model/linear plant pod elevation1 option 1/Coulomb_Friction_Model ==
  Torque : Inport
  velocity : Inport  Port=2
  velocity state : Inport  Port=3
  Abs2 : Abs  ZeroCross=off
  Gain : Gain
  Gain2 : Gain  Gain=1.1
  Hit Crossing : HitCross  ZeroCross=off
  MinMax : MinMax  Inputs=2
  Product1 : Product  RndMeth=Zero
  Product2 : Product  RndMeth=Zero
  Sign1 : Signum  ZeroCross=off
  Sign2 : Signum  ZeroCross=off
  Slip_T_friction : Constant  Value=fric_gear_motor_pod_elevation
  Stick_T_friction : Constant  Value=fric_gear_motor_pod_elevation
  Sw6 : Switch  Threshold=0.5  ZeroCross=off  SaturateOnIntegerOverflow=on  InputSameDT=on
  Friction_Torque : Outport
  reset velocity : Outport  Port=2
  wires:
  Torque/1 -> Sign1/1, Abs2/1
  Sw6/1 -> Friction_Torque/1
  Hit Crossing/1 -> reset velocity/1, Sw6/2
  Abs2/1 -> MinMax/2
  MinMax/1 -> Product2/1
  Product2/1 -> Sw6/1
  Product1/1 -> Sw6/3
  Stick_T_friction/1 -> Gain2/1
  Gain2/1 -> MinMax/1
  Sign2/1 -> Product1/2
  velocity/1 -> Sign2/1
  Sign1/1 -> Product2/2
  velocity state/1 -> Hit Crossing/1
  Slip_T_friction/1 -> Gain/1
  Gain/1 -> Product1/1

== system pod_elevation_model/linear plant pod elevation1 option 1/Coulomb_Friction_Model1 ==
  Torque : Inport
  velocity : Inport  Port=2
  velocity state : Inport  Port=3
  Abs2 : Abs  ZeroCross=off
  Gain : Gain
  Gain2 : Gain  Gain=1.1
  Hit Crossing : HitCross  ZeroCross=off
  MinMax : MinMax  Inputs=2
  Product1 : Product  RndMeth=Zero
  Product2 : Product  RndMeth=Zero
  Sign1 : Signum  ZeroCross=off
  Sign2 : Signum  ZeroCross=off
  Slip_T_friction : Constant  Value=fric_gear_motor_pod_elevation*0.7
  Stick_T_friction : Constant  Value=fric_gear_motor_pod_elevation*0.7
  Sw6 : Switch  Threshold=0.5  ZeroCross=off  SaturateOnIntegerOverflow=on  InputSameDT=on
  Friction_Torque : Outport
  reset velocity : Outport  Port=2
  wires:
  Torque/1 -> Sign1/1, Abs2/1
  Sw6/1 -> Friction_Torque/1
  Hit Crossing/1 -> reset velocity/1, Sw6/2
  Abs2/1 -> MinMax/2
  MinMax/1 -> Product2/1
  Product2/1 -> Sw6/1
  Product1/1 -> Sw6/3
  Stick_T_friction/1 -> Gain2/1
  Gain2/1 -> MinMax/1
  Sign2/1 -> Product1/2
  velocity/1 -> Sign2/1
  Sign1/1 -> Product2/2
  velocity state/1 -> Hit Crossing/1
  Slip_T_friction/1 -> Gain/1
  Gain/1 -> Product1/1
